simulink model "PV_Grid_Integration_VSC"  (R2025b)
settings: Solver=VariableStepAuto  StartTime=0.0  StopTime=1  MaxStep=1e-4  RelTol=1e-4
values from neighbouring files (symbols this model uses):
  Cdc = 278e-3    (= 0.278)    [PV_Grid_Integration_VSC_code.m]
  fg = 50    [PV_Grid_Integration_VSC_code.m]
  ki_pll = kp_pll/tau_pll    [PV_Grid_Integration_VSC_code.m]
  ki_v = 2.74e4    (= 27400)    [PV_Grid_Integration_VSC_code.m]
  kic = Rc/tauc    (= 0.95)    [PV_Grid_Integration_VSC_code.m]
  kip = 1/(ki_pq*tau_p)    [PV_Grid_Integration_VSC_code.m]
  kp_pll = xi_pll*2*omega_pll/Vpeak    [PV_Grid_Integration_VSC_code.m]
  kp_v = 123.5    [PV_Grid_Integration_VSC_code.m]
  kpc = Lc/tauc    (= 0.03031)    [PV_Grid_Integration_VSC_code.m]
  kpp = (tauc)/(ki_pq*tau_p)    [PV_Grid_Integration_VSC_code.m]
  Lc = 30.31e-6    (= 3.031e-05)    [PV_Grid_Integration_VSC_code.m]
  omega_pll = 2*pi*50    (= 314.159265359)    [PV_Grid_Integration_VSC_code.m]
  Rc = 0.95e-3    (= 0.00095)    [PV_Grid_Integration_VSC_code.m]
  Vdcn = 1200    [PV_Grid_Integration_VSC_code.m]
  Vpeak = Ucn*sqrt(2)/sqrt(3)    [PV_Grid_Integration_VSC_code.m]
libraries: spsControlledVoltageSourceLib x6, slpidlib x5, spsSeriesRLCBranchLib x4, spsControlledCurrentSourceLib x2, spsGroundLib x2, spsCurrentMeasurementLib x1, spsPower3phInstantaneousLib x1, spsThreePhaseVIMeasurementLib x1, spsVoltageMeasurementLib x1, sps_lib x1
settings Model: Creator=ibrahiml  LastModifiedBy=ibrahiml
settings DebuggingCC: AlgebraicLoopMsg=none

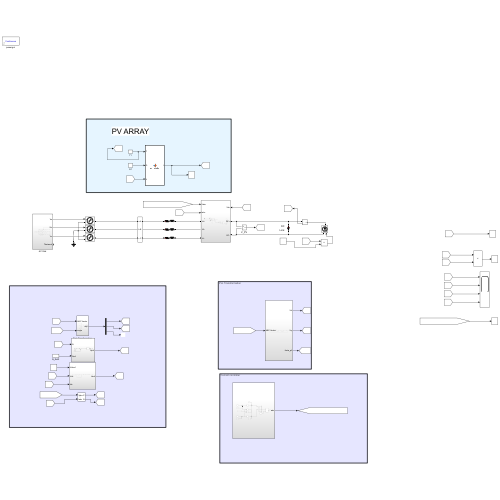
[thumbnail: Simulink's stored preview of the top-level diagram]
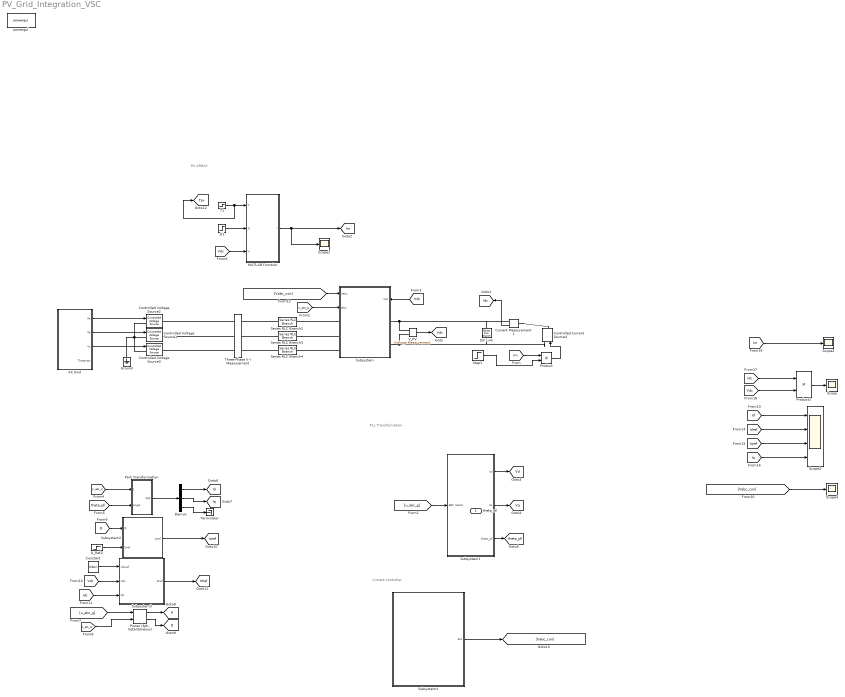
== system PV_Grid_Integration_VSC ==
  note: Current controller
  note: PLL Transformation
  note: PV ARRAY
  AC Grid : Subsystem
  Constant : Constant  Value=Vdcn
  Controlled Current Source3 : spsControlledCurrentSourceLib/Controlled Current Source  Initialize=on  Source_Type=DC  Amplitude=0  Phase=0  Frequency=0  Measurements=None
  Controlled Voltage Source1 : spsControlledVoltageSourceLib/Controlled Voltage Source  Initialize=off  Source_Type=AC  Amplitude=0  Phase=0  Frequency=0  Measurements=None
  Controlled Voltage Source2 : spsControlledVoltageSourceLib/Controlled Voltage Source  Initialize=off  Source_Type=AC  Amplitude=0  Phase=0  Frequency=0  Measurements=None
  Controlled Voltage Source3 : spsControlledVoltageSourceLib/Controlled Voltage Source  Initialize=off  Source_Type=AC  Amplitude=0  Phase=0  Frequency=0  Measurements=None
  Current Measurement1 : spsCurrentMeasurementLib/Current Measurement  PhasorSimulation=off  OutputType=Complex  PSBequivalent=0
  DC Link : spsSeriesRLCBranchLib/Series RLC Branch  LConnTagsString=__new0  RConnTagsString=__new0  BranchType=C  Resistance=1.0  Inductance=1.0  SetiL0=off  InitialCurrent=0  Capacitance=Cdc  Setx0=on  InitialVoltage=Vdcn  Measurements=None
  Demux : Demux  Outputs=3
  G1 : Step  Time=0.4  Before=800  After=580  SampleTime=0
  Ground : spsGroundLib/Ground  LConnTagsString=a
  MATLAB Function : MATLAB Function  TreatAsAtomicUnit=on
  Park Transformation : Subsystem
  "Power (3ph, Instantaneous)" : spsPower3phInstantaneousLib/Power (3ph, Instantaneous)
  Product : Product
  Product1 : Product
  Q_Ref2 : Step  Time=0.4  After=2.17e6  SampleTime=0
  Scope{,1..2,4} (4 alike) : Scope
      Scope settings: ActiveDisplayYMinimum=-539065.56359343883  ActiveDisplayYMaximum=3.8124909441925511E+6
      Scope1 settings: ActiveDisplayYMinimum=2165.3936795448935  ActiveDisplayYMaximum=4482.5713553620735
      Scope2 settings: ActiveDisplayYMinimum=1041.9775396767182  ActiveDisplayYMaximum=3525.4526268751893  DataLoggingVariableName=ScopeData3
      Scope4 settings: ActiveDisplayYMinimum=-747.60079786909239  ActiveDisplayYMaximum=827.75475751955958  DataLoggingVariableName=ScopeData5
  Scope3 : Scope  NumInputPorts=4
      settings: ActiveDisplayYMinimum=-2636.7120237029894  ActiveDisplayYMaximum=5175.2048904059839  DataLoggingVariableName=ScopeData4
  Series RLC Branch2 : spsSeriesRLCBranchLib/Series RLC Branch  LConnTagsString=__new0  RConnTagsString=__new0  BranchType=RL  Resistance=Rc  Inductance=Lc  SetiL0=off  InitialCurrent=0  Capacitance=1e-6  Setx0=off  InitialVoltage=0  Measurements=None
  Series RLC Branch3 : spsSeriesRLCBranchLib/Series RLC Branch  LConnTagsString=__new0  RConnTagsString=__new0  BranchType=RL  Resistance=Rc  Inductance=Lc  SetiL0=off  InitialCurrent=0  Capacitance=1e-6  Setx0=off  InitialVoltage=0  Measurements=None
  Series RLC Branch4 : spsSeriesRLCBranchLib/Series RLC Branch  LConnTagsString=__new0  RConnTagsString=__new0  BranchType=RL  Resistance=Rc  Inductance=Lc  SetiL0=off  InitialCurrent=0  Capacitance=1e-6  Setx0=off  InitialVoltage=0  Measurements=None
  Step1 : Step  Time=0.2  SampleTime=0
  Subsystem : Subsystem
      settings: PortSchema="{\"entries\":[{\"content\":{\"sides\":[{\"content\":{\"connectorIds\":[\"In1\",\"In2\",\"LConn1\",\"LConn2\",\"LConn3\"]},\"type\":\"ConnectorPlacement.EquallySpacedRectSide\",\"uuid\":\"119707c4-9f71-46f7-a757-ef0c87c2d619\"},{\"content\":{\"connectorIds\":[\"In3\",\"RConn1\",\"RConn2\"],\"side\":\"RIGHT\"},\"type\":\"ConnectorPlacement.EquallySpacedRectSide\",\"uuid\":\"ff6b650a-bef5-490f-a9c7-ea48b2f932e9\"},{\"content\":{\"side\":\"TOP\"},\"type\":\"ConnectorPlacement.EquallySpacedRectSide\",\"uuid\":\"2e01f8d1-159f-4140-ab20-4057d6ac11fa\"}]},\"type\":\"ConnectorPlacement.EquallySpacedConnector\",\"uuid\":\"bde8bbdd-2df2-490f-a66b-39e9c07d0c71\"}],\"packageUris\":[\"http://schema.mathworks.com/mf0/Connector/R2020b\"],\"version\":\"1.0\"}"
  Subsystem1 : Subsystem
  Subsystem2 : Subsystem
  Subsystem3 : Subsystem
  Subsystem4 : Subsystem
  T1 : Step  Time=0.2  Before=298  After=328  SampleTime=0
  Terminator : Terminator
  Three-Phase V-I Measurement : spsThreePhaseVIMeasurementLib/Three-Phase V-I Measurement  VoltageMeasurement=phase-to-ground  SetLabelV=on  LabelV=u_abc_g  Vpu=off  VpuLL=off  CurrentMeasurement=yes  SetLabelI=on  LabelI=i_abc_c  Ipu=off  Pbase=100e6  Vbase=500e3  OutputType=Complex  PhasorSimulation=off  PSBequivalent=0
  V_PV : spsVoltageMeasurementLib/Voltage Measurement  PhasorSimulation=off  OutputType=Complex  PSBequivalent=0
  powergui : sps_lib/powergui  Priority=1  SimulationMode=Continuous  SampleTime=50e-6  frequency=60  Iterations=50  frequencyindice=0  Pbase=100e6  ErrMax=1e-4  UnitsV=kV  UnitsW=MW  buscounter=0  FunctionMessages=off  echomessages=off  EnableUseOfTLC=off  CurrentSourceSwitches=off  DisableSnubberDevices=off  DisableRonSwitches=off  DisableVfSwitches=off  DisplayEquations=off  AutomaticDiscreteSolvers=off  SolverType=Tustin/Backward Euler (TBE)  Interpol=off  ExternalGateDelay=off  methode=off  Ts=100  x0status=blocks  SPID=on  SwTol=0  HookPort=off  NonlinearTolerance=1e-4  nMaxIteration=100  ContinueOnMaxIteration=off  RestoreLinks=warning  ResistiveCurrentMeasurement=off  Frange=[0:2:500]  Ylog=off  Xlog=on  ShowGrid=off  save=off  variable=ZData  structure=0  ZoomFFT=off  StartTime=0.0  cycles=1  DisplayStyle=1  fundamental=60  FreqAxis=off  MaxFrequency=1000  frequencyindicesteady=1  RmsSteady=1  display=off
  theta_pll : Outport
  tag scope: Id=global, Idc=global, Idref=global, Im=global, Iq=global, Iqref=global, P=global, Q=global, Tpv=global, Vd=global, Vdc=global, Vq=global, theta_pll=global
  wires:
  AC Grid/1(Va) -> Controlled Voltage Source2/1
  AC Grid/2(Vb) -> Controlled Voltage Source1/1
  AC Grid/3(Vc) -> Controlled Voltage Source3/1
  T1/1 -> [Tpv], MATLAB Function/1(T)
  [Vdc] -> MATLAB Function/3(V)
  MATLAB Function/1(I) -> [Im], Scope1/1
  G1/1 -> MATLAB Function/2(G)
  V_PV/1 -> [Vdc]
  Current Measurement1/1 -> [Idc]
  [u_abc_g] -> Subsystem1/1(ABC Vector)
  [i_abc_c] -> Subsystem/2(Iabc)
  [Vdc] -> Subsystem/3(Vdc)
  Subsystem1/1(Vd) -> [Vd]
  Subsystem1/3(theta_pll) -> [theta_pll]
  Subsystem1/2(Vq) -> [Vq]
  [i_abc_c] -> Park Transformation/1(ABC Vector)
  [theta_pll] -> Park Transformation/2(angle)
  Park Transformation/1(dq0) -> Demux/1
  Demux/1 -> [Id]
  Demux/2 -> [Iq]
  Demux/3 -> Terminator/1
  [u_abc_g] -> "Power (3ph, Instantaneous)"/1
  [i_abc_c] -> "Power (3ph, Instantaneous)"/2
  "Power (3ph, Instantaneous)"/1 -> [P]
  "Power (3ph, Instantaneous)"/2 -> [Q]
  [Q] -> Subsystem2/1(Q)
  Q_Ref2/1 -> Subsystem2/2(Qref)
  Constant/1 -> Subsystem3/1(Vdcref)
  [Vdc] -> Subsystem3/2(Vdc)
  [Idc] -> Subsystem3/3(Idc)
  Subsystem2/1(Iqref) -> [Iqref]
  Subsystem3/1(Idref) -> [Idref]
  Subsystem4/1(abc) -> [Vabc_con]
  [Vabc_con] -> Subsystem/1(Vabc)
  Product/1 -> Controlled Current Source3/1
  [Im] -> Product/1
  Step1/1 -> Product/2
  [Idc] -> Product1/1
  [Vdc] -> Product1/2
  Product1/1 -> Scope/1
  [Im] -> Scope2/1
  [Id] -> Scope3/1
  [Idref] -> Scope3/2
  [Iqref] -> Scope3/3
  [Iq] -> Scope3/4
  [Vabc_con] -> Scope4/1
  connections:
  Controlled Voltage Source2/LConn1 -- Ground/LConn1 -- Controlled Voltage Source3/LConn1 -- Controlled Voltage Source1/LConn1
  Three-Phase V-I Measurement/RConn1 -- Controlled Voltage Source2/RConn1
  Three-Phase V-I Measurement/RConn2 -- Controlled Voltage Source1/RConn1
  Three-Phase V-I Measurement/RConn3 -- Controlled Voltage Source3/RConn1
  Series RLC Branch2/LConn1 -- Three-Phase V-I Measurement/LConn1
  Series RLC Branch4/LConn1 -- Three-Phase V-I Measurement/LConn3
  Series RLC Branch3/LConn1 -- Three-Phase V-I Measurement/LConn2
  Subsystem/LConn1 -- Series RLC Branch2/RConn1
  Series RLC Branch3/RConn1 -- Subsystem/LConn2
  Subsystem/LConn3 -- Series RLC Branch4/RConn1
  V_PV/LConn1 -- Current Measurement1/RConn1 -- DC Link/LConn1 -- Subsystem/RConn1
  Subsystem/RConn2 -- Controlled Current Source3/LConn1 -- DC Link/RConn1 -- V_PV/LConn2
  Current Measurement1/LConn1 -- Controlled Current Source3/RConn1

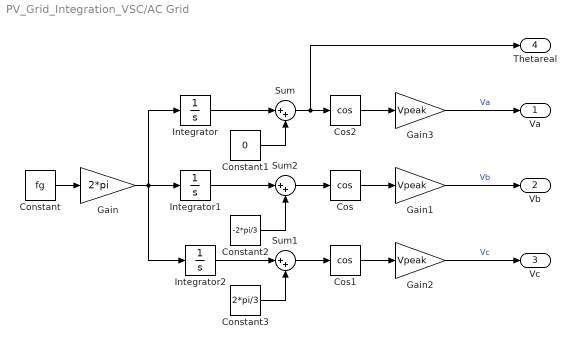
== system PV_Grid_Integration_VSC/AC Grid ==
  Constant : Constant  Value=fg
  Constant1 : Constant  Value=0
  Constant2 : Constant  Value=-2*pi/3
  Constant3 : Constant  Value=2*pi/3
  Cos : Trigonometry  Operator=cos
  Cos1 : Trigonometry  Operator=cos
  Cos2 : Trigonometry  Operator=cos
  Gain : Gain  Gain=2*pi
  Gain1 : Gain  Gain=Vpeak
  Gain2 : Gain  Gain=Vpeak
  Gain3 : Gain  Gain=Vpeak
  Integrator : Integrator
  Integrator1 : Integrator
  Integrator2 : Integrator
  Sum : Sum  Inputs=|++
  Sum1 : Sum  Inputs=|++
  Sum2 : Sum  Inputs=|++
  Va : Outport
  Vb : Outport  Port=2
  Vc : Outport  Port=3
  Thetareal : Outport  Port=4
  wires:
  Gain/1 -> Integrator/1, Integrator2/1, Integrator1/1
  Cos2/1 -> Gain3/1
  Constant2/1 -> Sum2/2
  Sum2/1 -> Cos/1
  Integrator/1 -> Sum/1
  Cos/1 -> Gain1/1
  Sum1/1 -> Cos1/1
  Constant/1 -> Gain/1
  Sum/1 -> Thetareal/1, Cos2/1
  Constant3/1 -> Sum1/2
  Gain3/1 -> Va/1  "Va"
  Integrator1/1 -> Sum2/1
  Constant1/1 -> Sum/2
  Integrator2/1 -> Sum1/1
  Cos1/1 -> Gain2/1
  Gain2/1 -> Vc/1  "Vc"
  Gain1/1 -> Vb/1  "Vb"

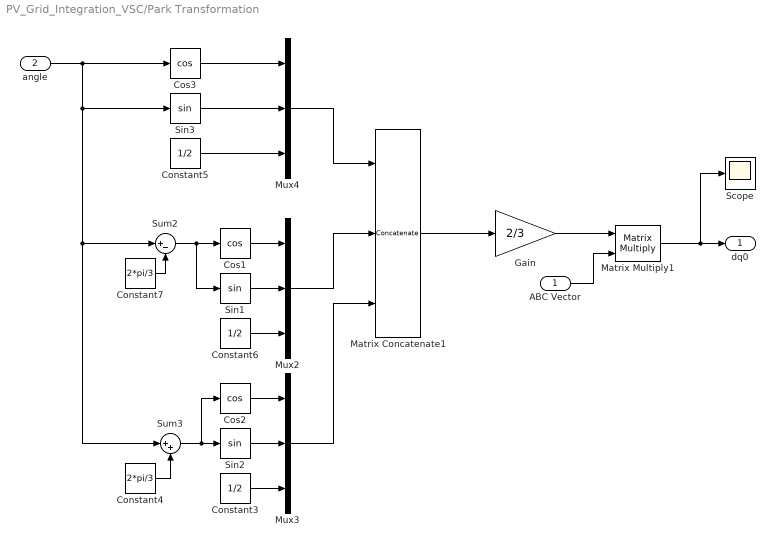
== system PV_Grid_Integration_VSC/Park Transformation ==
  ABC Vector : Inport
  angle : Inport  Port=2
  Constant3 : Constant  Value=1/2
  Constant4 : Constant  Value=2*pi/3
  Constant5 : Constant  Value=1/2
  Constant6 : Constant  Value=1/2
  Constant7 : Constant  Value=2*pi/3
  Cos1 : Trigonometry  Operator=cos
  Cos2 : Trigonometry  Operator=cos
  Cos3 : Trigonometry  Operator=cos
  Gain : Gain  Gain=2/3
  Matrix Concatenate1 : Concatenate  NumInputs=3  Mode=Multidimensional array  ConcatenateDimension=2
  Matrix Multiply1 : Product  Multiplication=Matrix(*)
  Mux2 : Mux  Inputs=3
  Mux3 : Mux  Inputs=3
  Mux4 : Mux  Inputs=3
  Scope : Scope
      settings: ActiveDisplayYMinimum=-2712.11745  ActiveDisplayYMaximum=5859.4781  DataLoggingVariableName=ScopeData2
  Sin1 : Trigonometry
  Sin2 : Trigonometry
  Sin3 : Trigonometry
  Sum2 : Sum  Inputs=|+-
  Sum3 : Sum  Inputs=|++
  dq0 : Outport
  wires:
  Cos2/1 -> Mux3/1
  Constant6/1 -> Mux2/3
  Gain/1 -> Matrix Multiply1/1
  angle/1 -> Cos3/1, Sin3/1, Sum3/1, Sum2/1
  Mux3/1 -> Matrix Concatenate1/3
  Mux4/1 -> Matrix Concatenate1/1
  Matrix Multiply1/1 -> Scope/1, dq0/1
  Constant5/1 -> Mux4/3
  Constant7/1 -> Sum2/2
  Sum2/1 -> Sin1/1, Cos1/1
  Sin1/1 -> Mux2/2
  Cos1/1 -> Mux2/1
  Sin2/1 -> Mux3/2
  Cos3/1 -> Mux4/1
  Sin3/1 -> Mux4/2
  Constant3/1 -> Mux3/3
  Constant4/1 -> Sum3/2
  Matrix Concatenate1/1 -> Gain/1
  Mux2/1 -> Matrix Concatenate1/2
  Sum3/1 -> Cos2/1, Sin2/1
  ABC Vector/1 -> Matrix Multiply1/2

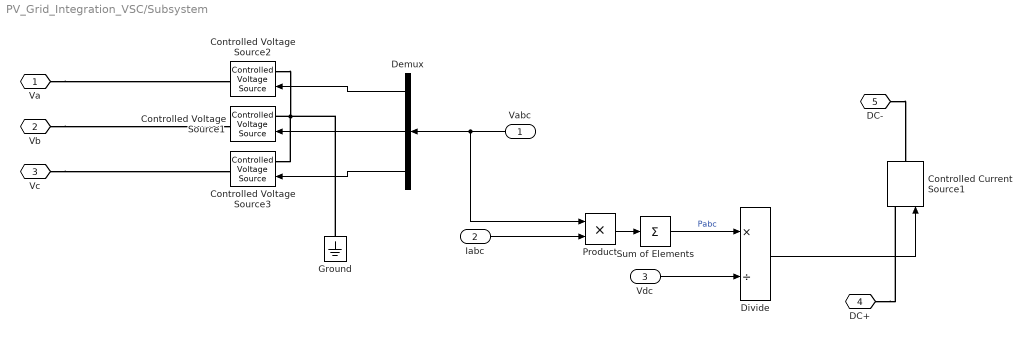
== system PV_Grid_Integration_VSC/Subsystem ==
  Vabc : Inport
  Iabc : Inport  Port=2
  Vdc : Inport  Port=3
  Controlled Current Source1 : spsControlledCurrentSourceLib/Controlled Current Source  Initialize=on  Source_Type=DC  Amplitude=0  Phase=0  Frequency=0  Measurements=None
  Controlled Voltage Source1 : spsControlledVoltageSourceLib/Controlled Voltage Source  Initialize=off  Source_Type=AC  Amplitude=0  Phase=0  Frequency=0  Measurements=None
  Controlled Voltage Source2 : spsControlledVoltageSourceLib/Controlled Voltage Source  Initialize=off  Source_Type=AC  Amplitude=0  Phase=0  Frequency=0  Measurements=None
  Controlled Voltage Source3 : spsControlledVoltageSourceLib/Controlled Voltage Source  Initialize=off  Source_Type=AC  Amplitude=0  Phase=0  Frequency=0  Measurements=None
  Demux : Demux  Outputs=3
  Divide : Product  Inputs=*/
  Ground : spsGroundLib/Ground  LConnTagsString=a
  Product : Product
  Sum of Elements : Sum  Inputs=+
  " Va" : PMIOPort  Side=Left
  " Vb" : PMIOPort  Port=2  Side=Left
  " Vc" : PMIOPort  Port=3  Side=Left
  " DC+" : PMIOPort  Port=4  Side=Right
  " DC-" : PMIOPort  Port=5  Side=Right
  wires:
  Demux/1 -> Controlled Voltage Source2/1
  Demux/2 -> Controlled Voltage Source1/1
  Demux/3 -> Controlled Voltage Source3/1
  Vabc/1 -> Product/1, Demux/1
  Iabc/1 -> Product/2
  Product/1 -> Sum of Elements/1
  Vdc/1 -> Divide/2
  Sum of Elements/1 -> Divide/1  "Pabc"
  Divide/1 -> Controlled Current Source1/1
  connections:
  Controlled Voltage Source2/LConn1 -- Ground/LConn1 -- Controlled Voltage Source3/LConn1 -- Controlled Voltage Source1/LConn1
  " Va"/RConn1 -- Controlled Voltage Source2/RConn1
  " Vb"/RConn1 -- Controlled Voltage Source1/RConn1
  " Vc"/RConn1 -- Controlled Voltage Source3/RConn1
  " DC-"/RConn1 -- Controlled Current Source1/RConn1
  " DC+"/RConn1 -- Controlled Current Source1/LConn1

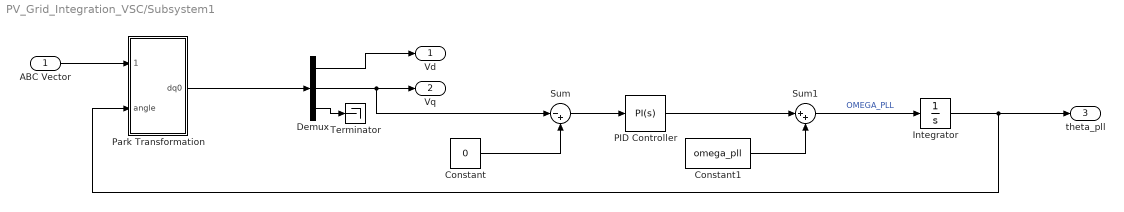
== system PV_Grid_Integration_VSC/Subsystem1 ==
  ABC Vector : Inport
  Constant : Constant  Value=0
  Constant1 : Constant  Value=omega_pll
  Demux : Demux  Outputs=3
  Integrator : Integrator
  PID Controller : slpidlib/PID Controller  Controller=PI  Form=Parallel  TimeDomain=Continuous-time  UseExternalTs=off  SampleTime=-1  IntegratorMethod=Forward Euler  FilterMethod=Forward Euler  ControllerParametersSource=internal  P=kp_pll  I=ki_pll  UseKiTs=off  D=0  UseExternalDerivativeSource=off  N=100  UseFilter=on  TunerSelectOption=Transfer Function Based (PID Tuner App)  InitialConditionSource=internal  InitialConditionForIntegrator=0  InitialConditionForFilter=0  DifferentiatorICPrevScaledInput=0  ExternalReset=none  TrackingMode=off  Kt=1  LimitOutput=off  SatLimitsSource=internal  UpperSaturationLimit=inf  LowerSaturationLimit=-inf  LinearizeAsGain=on  AntiWindupMode=none  Kb=1  LimitIntegrator=off  UpperIntegratorSaturationLimit=inf  LowerIntegratorSaturationLimit=-inf  POutMin=[]  POutMax=[]  IOutMin=[]  IOutMax=[]  DOutMin=[]  DOutMax=[]  NOutMin=[]  NOutMax=[]  SumOutMin=[]  SumOutMax=[]  SaturationOutMin=[]  SaturationOutMax=[]  PParamMin=[]  PParamMax=[]  IParamMin=[]  IParamMax=[]  DParamMin=[]  DParamMax=[]  NParamMin=[]  NParamMax=[]  KbParamMin=[]  KbParamMax=[]  KtParamMin=[]  KtParamMax=[]  KbOutMin=[]  KbOutMax=[]  KtOutMin=[]  KtOutMax=[]  IntegratorOutMin=[]  IntegratorOutMax=[]  FilterOutMin=[]  FilterOutMax=[]  SumI1OutMin=[]  SumI1OutMax=[]  SumI2OutMin=[]  SumI2OutMax=[]  SumI3OutMin=[]  SumI3OutMax=[]  SumI4OutMin=[]  SumI4OutMax=[]  SumDOutMin=[]  SumDOutMax=[]  DifferentiatorOutMin=[]  DifferentiatorOutMax=[]  FilterDiffOutCoefMin=[]  FilterDiffOutCoefMax=[]  ReciprocalOutMin=[]  ReciprocalOutMax=[]  SumDenOutMin=[]  SumDenOutMax=[]  SumNumOutMin=[]  SumNumOutMax=[]  DivideOutMin=[]  DivideOutMax=[]  UdiffTsProdOutMin=[]  UdiffTsProdOutMax=[]  NTsProdOutMin=[]  NTsProdOutMax=[]  UintegralTsProdOutMin=[]  UintegralTsProdOutMax=[]  UngainTsProdOutMin=[]  UngainTsProdOutMax=[]  ClampingZeroOutDataTypeStr=Inherit: Inherit via back propagation  ClampingZeroOutMin=[]  ClampingZeroOutMax=[]  FilterDenConstantOutDataTypeStr=Inherit: Inherit via back propagation  FilterDenConstantOutMin=[]  FilterDenConstantOutMax=[]  PCopyOutDataTypeStr=Inherit: Inherit via back propagation  PCopyOutMin=[]  PCopyOutMax=[]  NCopyOutDataTypeStr=Inherit: Inherit via back propagation  NCopyOutMin=[]  NCopyOutMax=[]  IntegratorContinuousStateAttributes=''  IntegratorStateMustResolveToSignalObject=off  IntegratorRTWStateStorageClass=Auto  FilterContinuousStateAttributes=''  FilterStateMustResolveToSignalObject=off  FilterRTWStateStorageClass=Auto  ParallelPVariant=InternalParameters  IdealPVariant=Disabled  IVariant=InternalParameters  DVariant=Disabled  IntegratorVariant=Continuous  SatVariant=Disabled  AWVariant=Passthrough  PCopyVariant=Disabled  TRVariant=Disabled  FdbkBlocksVariant=Forward  IdealPFdbkVariant=Disabled  SatFdbkVariant=Disabled  DerivativeFilterVariant=Disabled  NVariant=Disabled  NCopyVariant=Disabled_SignalSpec  FilterICVariant=Disabled  IntegratorICVariant=InternalICs  ExternalResetVariant=Disabled  TRSumVariant=Passthrough  SumFdbkVariant=Disabled  SumVariant=Sum_PI  TsampFilterVariant=InternalTs  TsampNgainVariant=Passthrough  TsampIntegralVariant=Disabled_SignalSpec  ExternalSaturationOutDataTypeStr=Inherit: Same as second input  DerivativeSourceVariant=Disabled  PreIntVariant=InternalPreInt
  Park Transformation : Subsystem
  Sum : Sum  Inputs=|-+
  Sum1 : Sum  Inputs=|++
  Terminator : Terminator
  Vd : Outport
  Vq : Outport  Port=2
  theta_pll : Outport  Port=3
  wires:
  Constant/1 -> Sum/2
  Demux/1 -> Vd/1
  Sum/1 -> PID Controller/1
  Park Transformation/1(dq0) -> Demux/1
  Demux/2 -> Vq/1, Sum/1
  Sum1/1 -> Integrator/1  "OMEGA_PLL"
  Demux/3 -> Terminator/1
  Constant1/1 -> Sum1/2
  PID Controller/1 -> Sum1/1
  ABC Vector/1 -> Park Transformation/1(ABC Vector)
  Integrator/1 -> Park Transformation/2(angle), theta_pll/1

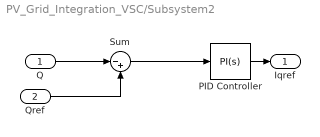
== system PV_Grid_Integration_VSC/Subsystem2 ==
  Q : Inport
  Qref : Inport  Port=2
  PID Controller : slpidlib/PID Controller  Controller=PI  Form=Parallel  TimeDomain=Continuous-time  UseExternalTs=off  SampleTime=-1  IntegratorMethod=Forward Euler  FilterMethod=Forward Euler  ControllerParametersSource=internal  P=kpp  I=kip  UseKiTs=off  D=0  UseExternalDerivativeSource=off  N=100  UseFilter=on  TunerSelectOption=Transfer Function Based (PID Tuner App)  InitialConditionSource=internal  InitialConditionForIntegrator=0  InitialConditionForFilter=0  DifferentiatorICPrevScaledInput=0  ExternalReset=none  TrackingMode=off  Kt=1  LimitOutput=off  SatLimitsSource=internal  UpperSaturationLimit=inf  LowerSaturationLimit=-inf  LinearizeAsGain=on  AntiWindupMode=none  Kb=1  LimitIntegrator=off  UpperIntegratorSaturationLimit=inf  LowerIntegratorSaturationLimit=-inf  POutMin=[]  POutMax=[]  IOutMin=[]  IOutMax=[]  DOutMin=[]  DOutMax=[]  NOutMin=[]  NOutMax=[]  SumOutMin=[]  SumOutMax=[]  SaturationOutMin=[]  SaturationOutMax=[]  PParamMin=[]  PParamMax=[]  IParamMin=[]  IParamMax=[]  DParamMin=[]  DParamMax=[]  NParamMin=[]  NParamMax=[]  KbParamMin=[]  KbParamMax=[]  KtParamMin=[]  KtParamMax=[]  KbOutMin=[]  KbOutMax=[]  KtOutMin=[]  KtOutMax=[]  IntegratorOutMin=[]  IntegratorOutMax=[]  FilterOutMin=[]  FilterOutMax=[]  SumI1OutMin=[]  SumI1OutMax=[]  SumI2OutMin=[]  SumI2OutMax=[]  SumI3OutMin=[]  SumI3OutMax=[]  SumI4OutMin=[]  SumI4OutMax=[]  SumDOutMin=[]  SumDOutMax=[]  DifferentiatorOutMin=[]  DifferentiatorOutMax=[]  FilterDiffOutCoefMin=[]  FilterDiffOutCoefMax=[]  ReciprocalOutMin=[]  ReciprocalOutMax=[]  SumDenOutMin=[]  SumDenOutMax=[]  SumNumOutMin=[]  SumNumOutMax=[]  DivideOutMin=[]  DivideOutMax=[]  UdiffTsProdOutMin=[]  UdiffTsProdOutMax=[]  NTsProdOutMin=[]  NTsProdOutMax=[]  UintegralTsProdOutMin=[]  UintegralTsProdOutMax=[]  UngainTsProdOutMin=[]  UngainTsProdOutMax=[]  ClampingZeroOutDataTypeStr=Inherit: Inherit via back propagation  ClampingZeroOutMin=[]  ClampingZeroOutMax=[]  FilterDenConstantOutDataTypeStr=Inherit: Inherit via back propagation  FilterDenConstantOutMin=[]  FilterDenConstantOutMax=[]  PCopyOutDataTypeStr=Inherit: Inherit via back propagation  PCopyOutMin=[]  PCopyOutMax=[]  NCopyOutDataTypeStr=Inherit: Inherit via back propagation  NCopyOutMin=[]  NCopyOutMax=[]  IntegratorContinuousStateAttributes=''  IntegratorStateMustResolveToSignalObject=off  IntegratorRTWStateStorageClass=Auto  FilterContinuousStateAttributes=''  FilterStateMustResolveToSignalObject=off  FilterRTWStateStorageClass=Auto  ParallelPVariant=InternalParameters  IdealPVariant=Disabled  IVariant=InternalParameters  DVariant=Disabled  IntegratorVariant=Continuous  SatVariant=Disabled  AWVariant=Passthrough  PCopyVariant=Disabled  TRVariant=Disabled  FdbkBlocksVariant=Forward  IdealPFdbkVariant=Disabled  SatFdbkVariant=Disabled  DerivativeFilterVariant=Disabled  NVariant=Disabled  NCopyVariant=Disabled_SignalSpec  FilterICVariant=Disabled  IntegratorICVariant=InternalICs  ExternalResetVariant=Disabled  TRSumVariant=Passthrough  SumFdbkVariant=Disabled  SumVariant=Sum_PI  TsampFilterVariant=InternalTs  TsampNgainVariant=Passthrough  TsampIntegralVariant=Disabled_SignalSpec  ExternalSaturationOutDataTypeStr=Inherit: Same as second input  DerivativeSourceVariant=Disabled  PreIntVariant=InternalPreInt
  Sum : Sum  Inputs=|-+
  Iqref : Outport
  wires:
  Qref/1 -> Sum/2
  Sum/1 -> PID Controller/1
  PID Controller/1 -> Iqref/1
  Q/1 -> Sum/1

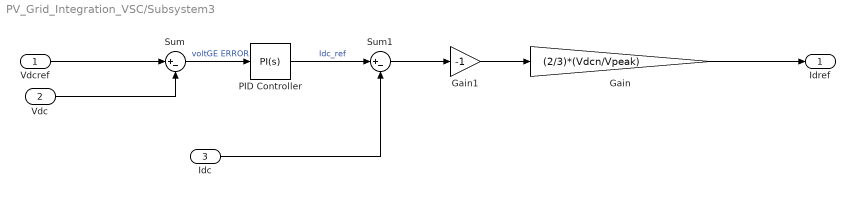
== system PV_Grid_Integration_VSC/Subsystem3 ==
  Vdcref : Inport
  Vdc : Inport  Port=2
  Idc : Inport  Port=3
  Gain : Gain  Gain=(2/3)*(Vdcn/Vpeak)
  Gain1 : Gain  Gain=-1
  PID Controller : slpidlib/PID Controller  Controller=PI  Form=Parallel  TimeDomain=Continuous-time  UseExternalTs=off  SampleTime=-1  IntegratorMethod=Forward Euler  FilterMethod=Forward Euler  ControllerParametersSource=internal  P=kp_v  I=ki_v  UseKiTs=off  D=0  UseExternalDerivativeSource=off  N=100  UseFilter=on  TunerSelectOption=Transfer Function Based (PID Tuner App)  InitialConditionSource=internal  InitialConditionForIntegrator=0  InitialConditionForFilter=0  DifferentiatorICPrevScaledInput=0  ExternalReset=none  TrackingMode=off  Kt=1  LimitOutput=off  SatLimitsSource=internal  UpperSaturationLimit=inf  LowerSaturationLimit=-inf  LinearizeAsGain=on  AntiWindupMode=none  Kb=1  LimitIntegrator=off  UpperIntegratorSaturationLimit=inf  LowerIntegratorSaturationLimit=-inf  POutMin=[]  POutMax=[]  IOutMin=[]  IOutMax=[]  DOutMin=[]  DOutMax=[]  NOutMin=[]  NOutMax=[]  SumOutMin=[]  SumOutMax=[]  SaturationOutMin=[]  SaturationOutMax=[]  PParamMin=[]  PParamMax=[]  IParamMin=[]  IParamMax=[]  DParamMin=[]  DParamMax=[]  NParamMin=[]  NParamMax=[]  KbParamMin=[]  KbParamMax=[]  KtParamMin=[]  KtParamMax=[]  KbOutMin=[]  KbOutMax=[]  KtOutMin=[]  KtOutMax=[]  IntegratorOutMin=[]  IntegratorOutMax=[]  FilterOutMin=[]  FilterOutMax=[]  SumI1OutMin=[]  SumI1OutMax=[]  SumI2OutMin=[]  SumI2OutMax=[]  SumI3OutMin=[]  SumI3OutMax=[]  SumI4OutMin=[]  SumI4OutMax=[]  SumDOutMin=[]  SumDOutMax=[]  DifferentiatorOutMin=[]  DifferentiatorOutMax=[]  FilterDiffOutCoefMin=[]  FilterDiffOutCoefMax=[]  ReciprocalOutMin=[]  ReciprocalOutMax=[]  SumDenOutMin=[]  SumDenOutMax=[]  SumNumOutMin=[]  SumNumOutMax=[]  DivideOutMin=[]  DivideOutMax=[]  UdiffTsProdOutMin=[]  UdiffTsProdOutMax=[]  NTsProdOutMin=[]  NTsProdOutMax=[]  UintegralTsProdOutMin=[]  UintegralTsProdOutMax=[]  UngainTsProdOutMin=[]  UngainTsProdOutMax=[]  ClampingZeroOutDataTypeStr=Inherit: Inherit via back propagation  ClampingZeroOutMin=[]  ClampingZeroOutMax=[]  FilterDenConstantOutDataTypeStr=Inherit: Inherit via back propagation  FilterDenConstantOutMin=[]  FilterDenConstantOutMax=[]  PCopyOutDataTypeStr=Inherit: Inherit via back propagation  PCopyOutMin=[]  PCopyOutMax=[]  NCopyOutDataTypeStr=Inherit: Inherit via back propagation  NCopyOutMin=[]  NCopyOutMax=[]  IntegratorContinuousStateAttributes=''  IntegratorStateMustResolveToSignalObject=off  IntegratorRTWStateStorageClass=Auto  FilterContinuousStateAttributes=''  FilterStateMustResolveToSignalObject=off  FilterRTWStateStorageClass=Auto  ParallelPVariant=InternalParameters  IdealPVariant=Disabled  IVariant=InternalParameters  DVariant=Disabled  IntegratorVariant=Continuous  SatVariant=Disabled  AWVariant=Passthrough  PCopyVariant=Disabled  TRVariant=Disabled  FdbkBlocksVariant=Forward  IdealPFdbkVariant=Disabled  SatFdbkVariant=Disabled  DerivativeFilterVariant=Disabled  NVariant=Disabled  NCopyVariant=Disabled_SignalSpec  FilterICVariant=Disabled  IntegratorICVariant=InternalICs  ExternalResetVariant=Disabled  TRSumVariant=Passthrough  SumFdbkVariant=Disabled  SumVariant=Sum_PI  TsampFilterVariant=InternalTs  TsampNgainVariant=Passthrough  TsampIntegralVariant=Disabled_SignalSpec  ExternalSaturationOutDataTypeStr=Inherit: Same as second input  DerivativeSourceVariant=Disabled  PreIntVariant=InternalPreInt
  Sum : Sum  Inputs=|+-
  Sum1 : Sum  Inputs=|+-
  Idref : Outport
  wires:
  Idc/1 -> Sum1/2
  Sum1/1 -> Gain1/1
  Vdc/1 -> Sum/2
  Vdcref/1 -> Sum/1
  PID Controller/1 -> Sum1/1  "Idc_ref"
  Gain/1 -> Idref/1
  Gain1/1 -> Gain/1
  Sum/1 -> PID Controller/1  "voltGE ERROR"

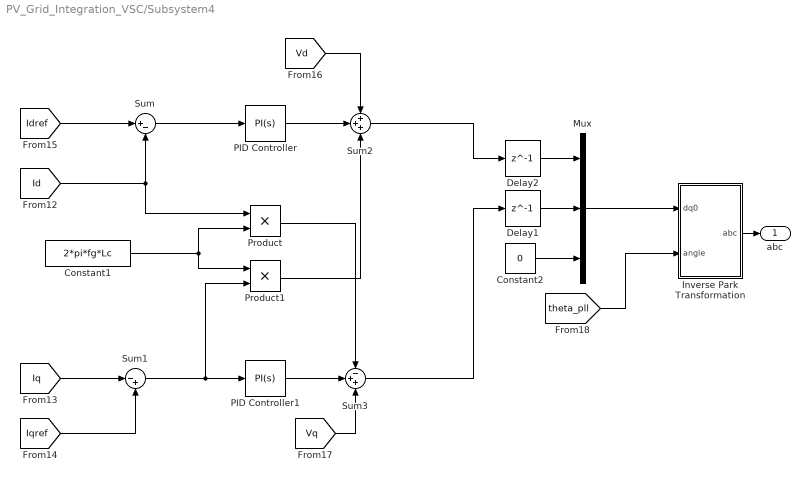
== system PV_Grid_Integration_VSC/Subsystem4 ==
  Constant1 : Constant  Value=2*pi*fg*Lc
  Constant2 : Constant  Value=0
  Delay1 : Delay  DelayLength=1  InputProcessing=Columns as channels (frame based)
  Delay2 : Delay  DelayLength=1  InputProcessing=Columns as channels (frame based)
  Inverse Park Transformation : Subsystem
  Mux : Mux  Inputs=3
  PID Controller : slpidlib/PID Controller  Controller=PI  Form=Parallel  TimeDomain=Continuous-time  UseExternalTs=off  SampleTime=-1  IntegratorMethod=Forward Euler  FilterMethod=Forward Euler  ControllerParametersSource=internal  P=kpc  I=kic  UseKiTs=off  D=0  UseExternalDerivativeSource=off  N=100  UseFilter=on  TunerSelectOption=Transfer Function Based (PID Tuner App)  InitialConditionSource=internal  InitialConditionForIntegrator=0  InitialConditionForFilter=0  DifferentiatorICPrevScaledInput=0  ExternalReset=none  TrackingMode=off  Kt=1  LimitOutput=off  SatLimitsSource=internal  UpperSaturationLimit=inf  LowerSaturationLimit=-inf  LinearizeAsGain=on  AntiWindupMode=none  Kb=1  LimitIntegrator=off  UpperIntegratorSaturationLimit=inf  LowerIntegratorSaturationLimit=-inf  POutMin=[]  POutMax=[]  IOutMin=[]  IOutMax=[]  DOutMin=[]  DOutMax=[]  NOutMin=[]  NOutMax=[]  SumOutMin=[]  SumOutMax=[]  SaturationOutMin=[]  SaturationOutMax=[]  PParamMin=[]  PParamMax=[]  IParamMin=[]  IParamMax=[]  DParamMin=[]  DParamMax=[]  NParamMin=[]  NParamMax=[]  KbParamMin=[]  KbParamMax=[]  KtParamMin=[]  KtParamMax=[]  KbOutMin=[]  KbOutMax=[]  KtOutMin=[]  KtOutMax=[]  IntegratorOutMin=[]  IntegratorOutMax=[]  FilterOutMin=[]  FilterOutMax=[]  SumI1OutMin=[]  SumI1OutMax=[]  SumI2OutMin=[]  SumI2OutMax=[]  SumI3OutMin=[]  SumI3OutMax=[]  SumI4OutMin=[]  SumI4OutMax=[]  SumDOutMin=[]  SumDOutMax=[]  DifferentiatorOutMin=[]  DifferentiatorOutMax=[]  FilterDiffOutCoefMin=[]  FilterDiffOutCoefMax=[]  ReciprocalOutMin=[]  ReciprocalOutMax=[]  SumDenOutMin=[]  SumDenOutMax=[]  SumNumOutMin=[]  SumNumOutMax=[]  DivideOutMin=[]  DivideOutMax=[]  UdiffTsProdOutMin=[]  UdiffTsProdOutMax=[]  NTsProdOutMin=[]  NTsProdOutMax=[]  UintegralTsProdOutMin=[]  UintegralTsProdOutMax=[]  UngainTsProdOutMin=[]  UngainTsProdOutMax=[]  ClampingZeroOutDataTypeStr=Inherit: Inherit via back propagation  ClampingZeroOutMin=[]  ClampingZeroOutMax=[]  FilterDenConstantOutDataTypeStr=Inherit: Inherit via back propagation  FilterDenConstantOutMin=[]  FilterDenConstantOutMax=[]  PCopyOutDataTypeStr=Inherit: Inherit via back propagation  PCopyOutMin=[]  PCopyOutMax=[]  NCopyOutDataTypeStr=Inherit: Inherit via back propagation  NCopyOutMin=[]  NCopyOutMax=[]  IntegratorContinuousStateAttributes=''  IntegratorStateMustResolveToSignalObject=off  IntegratorRTWStateStorageClass=Auto  FilterContinuousStateAttributes=''  FilterStateMustResolveToSignalObject=off  FilterRTWStateStorageClass=Auto  ParallelPVariant=InternalParameters  IdealPVariant=Disabled  IVariant=InternalParameters  DVariant=Disabled  IntegratorVariant=Continuous  SatVariant=Disabled  AWVariant=Passthrough  PCopyVariant=Disabled  TRVariant=Disabled  FdbkBlocksVariant=Forward  IdealPFdbkVariant=Disabled  SatFdbkVariant=Disabled  DerivativeFilterVariant=Disabled  NVariant=Disabled  NCopyVariant=Disabled_SignalSpec  FilterICVariant=Disabled  IntegratorICVariant=InternalICs  ExternalResetVariant=Disabled  TRSumVariant=Passthrough  SumFdbkVariant=Disabled  SumVariant=Sum_PI  TsampFilterVariant=InternalTs  TsampNgainVariant=Passthrough  TsampIntegralVariant=Disabled_SignalSpec  ExternalSaturationOutDataTypeStr=Inherit: Same as second input  DerivativeSourceVariant=Disabled  PreIntVariant=InternalPreInt
  PID Controller1 : slpidlib/PID Controller  Controller=PI  Form=Parallel  TimeDomain=Continuous-time  UseExternalTs=off  SampleTime=-1  IntegratorMethod=Forward Euler  FilterMethod=Forward Euler  ControllerParametersSource=internal  P=kpc  I=kic  UseKiTs=off  D=0  UseExternalDerivativeSource=off  N=100  UseFilter=on  TunerSelectOption=Transfer Function Based (PID Tuner App)  InitialConditionSource=internal  InitialConditionForIntegrator=0  InitialConditionForFilter=0  DifferentiatorICPrevScaledInput=0  ExternalReset=none  TrackingMode=off  Kt=1  LimitOutput=off  SatLimitsSource=internal  UpperSaturationLimit=inf  LowerSaturationLimit=-inf  LinearizeAsGain=on  AntiWindupMode=none  Kb=1  LimitIntegrator=off  UpperIntegratorSaturationLimit=inf  LowerIntegratorSaturationLimit=-inf  POutMin=[]  POutMax=[]  IOutMin=[]  IOutMax=[]  DOutMin=[]  DOutMax=[]  NOutMin=[]  NOutMax=[]  SumOutMin=[]  SumOutMax=[]  SaturationOutMin=[]  SaturationOutMax=[]  PParamMin=[]  PParamMax=[]  IParamMin=[]  IParamMax=[]  DParamMin=[]  DParamMax=[]  NParamMin=[]  NParamMax=[]  KbParamMin=[]  KbParamMax=[]  KtParamMin=[]  KtParamMax=[]  KbOutMin=[]  KbOutMax=[]  KtOutMin=[]  KtOutMax=[]  IntegratorOutMin=[]  IntegratorOutMax=[]  FilterOutMin=[]  FilterOutMax=[]  SumI1OutMin=[]  SumI1OutMax=[]  SumI2OutMin=[]  SumI2OutMax=[]  SumI3OutMin=[]  SumI3OutMax=[]  SumI4OutMin=[]  SumI4OutMax=[]  SumDOutMin=[]  SumDOutMax=[]  DifferentiatorOutMin=[]  DifferentiatorOutMax=[]  FilterDiffOutCoefMin=[]  FilterDiffOutCoefMax=[]  ReciprocalOutMin=[]  ReciprocalOutMax=[]  SumDenOutMin=[]  SumDenOutMax=[]  SumNumOutMin=[]  SumNumOutMax=[]  DivideOutMin=[]  DivideOutMax=[]  UdiffTsProdOutMin=[]  UdiffTsProdOutMax=[]  NTsProdOutMin=[]  NTsProdOutMax=[]  UintegralTsProdOutMin=[]  UintegralTsProdOutMax=[]  UngainTsProdOutMin=[]  UngainTsProdOutMax=[]  ClampingZeroOutDataTypeStr=Inherit: Inherit via back propagation  ClampingZeroOutMin=[]  ClampingZeroOutMax=[]  FilterDenConstantOutDataTypeStr=Inherit: Inherit via back propagation  FilterDenConstantOutMin=[]  FilterDenConstantOutMax=[]  PCopyOutDataTypeStr=Inherit: Inherit via back propagation  PCopyOutMin=[]  PCopyOutMax=[]  NCopyOutDataTypeStr=Inherit: Inherit via back propagation  NCopyOutMin=[]  NCopyOutMax=[]  IntegratorContinuousStateAttributes=''  IntegratorStateMustResolveToSignalObject=off  IntegratorRTWStateStorageClass=Auto  FilterContinuousStateAttributes=''  FilterStateMustResolveToSignalObject=off  FilterRTWStateStorageClass=Auto  ParallelPVariant=InternalParameters  IdealPVariant=Disabled  IVariant=InternalParameters  DVariant=Disabled  IntegratorVariant=Continuous  SatVariant=Disabled  AWVariant=Passthrough  PCopyVariant=Disabled  TRVariant=Disabled  FdbkBlocksVariant=Forward  IdealPFdbkVariant=Disabled  SatFdbkVariant=Disabled  DerivativeFilterVariant=Disabled  NVariant=Disabled  NCopyVariant=Disabled_SignalSpec  FilterICVariant=Disabled  IntegratorICVariant=InternalICs  ExternalResetVariant=Disabled  TRSumVariant=Passthrough  SumFdbkVariant=Disabled  SumVariant=Sum_PI  TsampFilterVariant=InternalTs  TsampNgainVariant=Passthrough  TsampIntegralVariant=Disabled_SignalSpec  ExternalSaturationOutDataTypeStr=Inherit: Same as second input  DerivativeSourceVariant=Disabled  PreIntVariant=InternalPreInt
  Product : Product
  Product1 : Product
  Sum : Sum  Inputs=|+-
  Sum1 : Sum  Inputs=|-+
  Sum2 : Sum  Inputs=+++
  Sum3 : Sum  Inputs=-++
  abc : Outport
  wires:
  Mux/1 -> Inverse Park Transformation/1(dq0)
  Sum2/1 -> Delay2/1
  [Id] -> Sum/2, Product/1
  Constant1/1 -> Product1/1, Product/2
  [Idref] -> Sum/1
  Constant2/1 -> Mux/3
  Sum/1 -> PID Controller/1
  [theta_pll] -> Inverse Park Transformation/2(angle)
  Sum1/1 -> Product1/2, PID Controller1/1
  PID Controller/1 -> Sum2/2
  [Iq] -> Sum1/1
  [Vq] -> Sum3/3
  Delay2/1 -> Mux/1
  Inverse Park Transformation/1(abc) -> abc/1
  [Vd] -> Sum2/1
  [Iqref] -> Sum1/2
  Sum3/1 -> Delay1/1
  Delay1/1 -> Mux/2
  Product/1 -> Sum3/1
  PID Controller1/1 -> Sum3/2
  Product1/1 -> Sum2/3

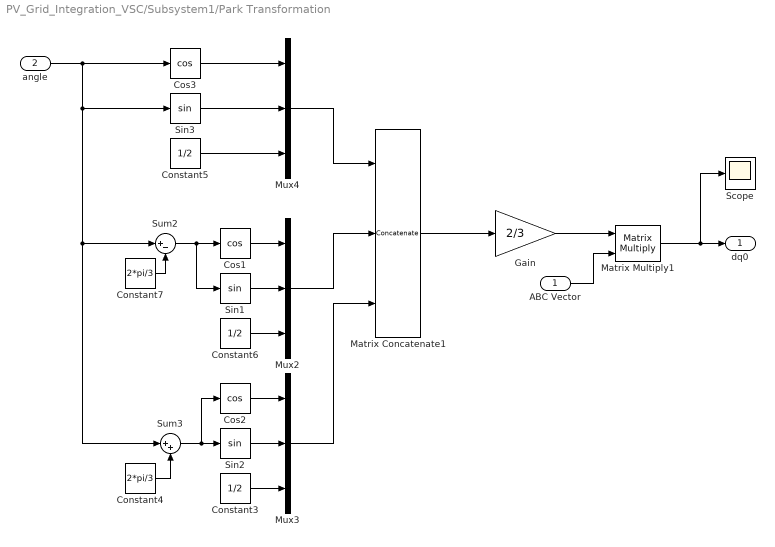
== system PV_Grid_Integration_VSC/Subsystem1/Park Transformation ==
  ABC Vector : Inport
  angle : Inport  Port=2
  Constant3 : Constant  Value=1/2
  Constant4 : Constant  Value=2*pi/3
  Constant5 : Constant  Value=1/2
  Constant6 : Constant  Value=1/2
  Constant7 : Constant  Value=2*pi/3
  Cos1 : Trigonometry  Operator=cos
  Cos2 : Trigonometry  Operator=cos
  Cos3 : Trigonometry  Operator=cos
  Gain : Gain  Gain=2/3
  Matrix Concatenate1 : Concatenate  NumInputs=3  Mode=Multidimensional array  ConcatenateDimension=2
  Matrix Multiply1 : Product  Multiplication=Matrix(*)
  Mux2 : Mux  Inputs=3
  Mux3 : Mux  Inputs=3
  Mux4 : Mux  Inputs=3
  Scope : Scope
      settings: ActiveDisplayYMinimum=-2712.11745  ActiveDisplayYMaximum=5859.4781  DataLoggingVariableName=ScopeData2
  Sin1 : Trigonometry
  Sin2 : Trigonometry
  Sin3 : Trigonometry
  Sum2 : Sum  Inputs=|+-
  Sum3 : Sum  Inputs=|++
  dq0 : Outport
  wires:
  Cos2/1 -> Mux3/1
  Constant6/1 -> Mux2/3
  Gain/1 -> Matrix Multiply1/1
  angle/1 -> Cos3/1, Sin3/1, Sum3/1, Sum2/1
  Mux3/1 -> Matrix Concatenate1/3
  Mux4/1 -> Matrix Concatenate1/1
  Matrix Multiply1/1 -> Scope/1, dq0/1
  Constant5/1 -> Mux4/3
  Constant7/1 -> Sum2/2
  Sum2/1 -> Sin1/1, Cos1/1
  Sin1/1 -> Mux2/2
  Cos1/1 -> Mux2/1
  Sin2/1 -> Mux3/2
  Cos3/1 -> Mux4/1
  Sin3/1 -> Mux4/2
  Constant3/1 -> Mux3/3
  Constant4/1 -> Sum3/2
  Matrix Concatenate1/1 -> Gain/1
  Mux2/1 -> Matrix Concatenate1/2
  Sum3/1 -> Cos2/1, Sin2/1
  ABC Vector/1 -> Matrix Multiply1/2

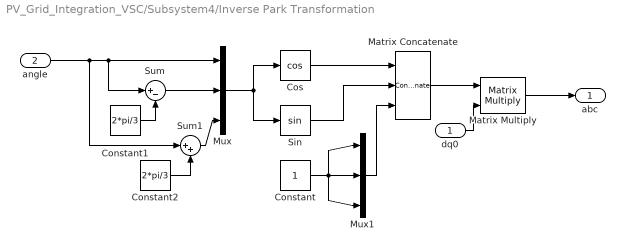
== system PV_Grid_Integration_VSC/Subsystem4/Inverse Park Transformation ==
  dq0 : Inport
  angle : Inport  Port=2
  Constant : Constant
  Constant1 : Constant  Value=2*pi/3
  Constant2 : Constant  Value=2*pi/3
  Cos : Trigonometry  Operator=cos
  Matrix Concatenate : Concatenate  NumInputs=3  Mode=Multidimensional array  ConcatenateDimension=2
  Matrix Multiply : Product  Multiplication=Matrix(*)
  Mux : Mux  Inputs=3
  Mux1 : Mux  Inputs=3
  Sin : Trigonometry
  Sum : Sum  Inputs=|+-
  Sum1 : Sum  Inputs=|++
  abc : Outport
  wires:
  dq0/1 -> Matrix Multiply/2
  Sum/1 -> Mux/2
  Constant/1 -> Mux1/3, Mux1/1, Mux1/2
  Mux/1 -> Cos/1, Sin/1
  Constant2/1 -> Sum1/2
  Sin/1 -> Matrix Concatenate/2
  Cos/1 -> Matrix Concatenate/1
  Mux1/1 -> Matrix Concatenate/3
  angle/1 -> Sum/1, Mux/1, Sum1/1
  Matrix Concatenate/1 -> Matrix Multiply/1
  Sum1/1 -> Mux/3
  Constant1/1 -> Sum/2
  Matrix Multiply/1 -> abc/1

== matlab function PV_Grid_Integration_VSC/MATLAB Function ==
  data: T input; G input; V input; I output
function I  = pv_diode(T, G, V)
% Full single diode PV model WITH Rs*I inside exp(), solved using Newton.
% Inputs:
%   T  - temperature [K]
%   G  - irradiance [W/m^2]
%   V  - PV array voltage [V]

    % ---- PV Parameters (Your values) ----
    Isc = 8.21;
    Voc = 32.9;
    Kv  = -0.123;
    Ki  = 0.0032;
    Rp  = 415.405;
    Rs  = 0.221;
    a   = 1.3;
    Ns  = 54;
    Tn  = 25 + 273.15;
    Gn  = 1000;
    kq  = 1.38e-23 / 1.6e-19;
    ser = 45;
    par = 690;

    % ---- 1) Photocurrent ----
    Ipv = ( (Isc*(Rp + Rs)/Rp) + Ki*(T - Tn) ) * (G / Gn);

    % ---- 2) Saturation current ----
    Vt_cell = a * kq * Tn;      
    den0 = Ns * Vt_cell;
    I0 = (Isc + Ki*(T - Tn)) / ( exp((Voc + Kv*(T - Tn))/den0) - 1 );

    % ---- 3) Solve implicit equation using Newton iteration ----
    Vcell = V / ser;
    I = Ipv * par;   % Initial guess: short-circuit approx

    for k = 1:5
        term = Vcell + (Rs/par)*I;
        exp_term = exp(term / den0);

        f = par*(Ipv - I0*(exp_term - 1) - term/Rp) - I;

        % Derivative df/dI
        df = par * ( ...
                -I0 * (exp_term) * (Rs/(par*den0)) ...
                - (Rs/(par*Rp)) ...
            ) - 1;

        I = I - f/df;
    end

end
